simulink subsystem "template_MPC_offline_traj_shared_subsystem_MCP2_opti_qrqp"  (R2023b)
settings: Solver=VariableStepAuto  StartTime=0.0  StopTime=10.0  RelTol=1e-3
undefined symbols (not defined in the file): param_MPC2_qrqp_opti, param_MPC2_qrqp_opti_traj_data, param_weight_MPC2_qrqp_opti
settings Model: Creator=emu  LastModifiedBy=emu

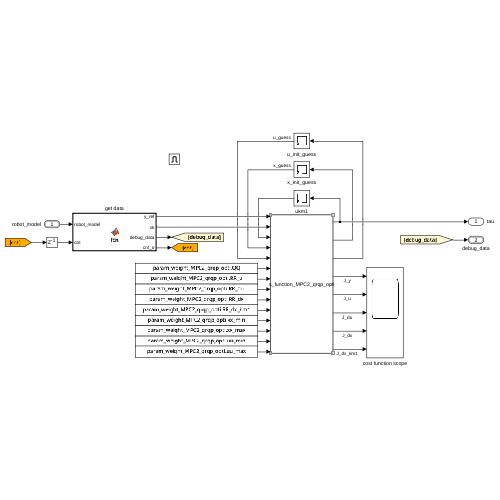
[thumbnail: Simulink's stored preview of the top-level diagram]
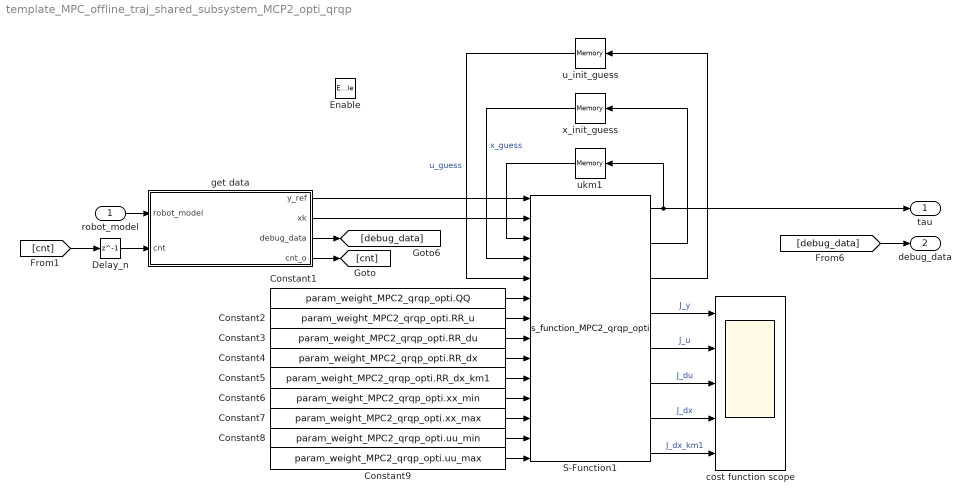
== system template_MPC_offline_traj_shared_subsystem_MCP2_opti_qrqp ==
  robot_model : Inport  OutDataTypeStr=Bus: robot_model
  Enable : EnablePort
  Constant1 : Constant  Value=param_weight_MPC2_qrqp_opti.QQ
  Constant2 : Constant  Value=param_weight_MPC2_qrqp_opti.RR_u
  Constant3 : Constant  Value=param_weight_MPC2_qrqp_opti.RR_du
  Constant4 : Constant  Value=param_weight_MPC2_qrqp_opti.RR_dx
  Constant5 : Constant  Value=param_weight_MPC2_qrqp_opti.RR_dx_km1
  Constant6 : Constant  Value=param_weight_MPC2_qrqp_opti.xx_min
  Constant7 : Constant  Value=param_weight_MPC2_qrqp_opti.xx_max
  Constant8 : Constant  Value=param_weight_MPC2_qrqp_opti.uu_min
  Constant9 : Constant  Value=param_weight_MPC2_qrqp_opti.uu_max
  Delay_n : Delay  DelayLength=1  InitialCondition=1
  S-Function1 : S-Function  FunctionName=s_function_MPC2_qrqp_opti  SFunctionModules='MPC2_qrqp_opti'  SFunctionDeploymentMode=off  EnableBusSupport=off
  cost function scope : Scope  NumInputPorts=5
  get data : MATLAB Function  TreatAsAtomicUnit=on
  u_init_guess : Memory  InitialCondition=param_MPC2_qrqp_opti.u_init_guess
  ukm1 : Memory  InitialCondition=param_MPC2_qrqp_opti.u_init_guess(:,1)
  x_init_guess : Memory  InitialCondition=param_MPC2_qrqp_opti.x_init_guess
  tau : Outport
  debug_data : Outport  Port=2  OutDataTypeStr=Bus: debug_data_bus
  wires:
  get data/1(y_ref) -> S-Function1/1
  S-Function1/6 -> cost function scope/3  "J_du"
  S-Function1/1 -> ukm1/1, tau/1
  ukm1/1 -> S-Function1/3
  x_init_guess/1 -> S-Function1/4  "x_guess"
  S-Function1/2 -> x_init_guess/1
  S-Function1/8 -> cost function scope/5  "J_dx_km1"
  S-Function1/3 -> u_init_guess/1
  get data/2(xk) -> S-Function1/2
  Constant4/1 -> S-Function1/9
  [cnt] -> Delay_n/1
  get data/4(cnt_o) -> [cnt]
  S-Function1/4 -> cost function scope/1  "J_y"
  Constant6/1 -> S-Function1/11
  S-Function1/5 -> cost function scope/2  "J_u"
  [debug_data] -> debug_data/1
  Constant9/1 -> S-Function1/14
  Delay_n/1 -> get data/2(cnt)
  u_init_guess/1 -> S-Function1/5  "u_guess"
  Constant8/1 -> S-Function1/13
  Constant3/1 -> S-Function1/8
  Constant5/1 -> S-Function1/10
  Constant2/1 -> S-Function1/7
  Constant1/1 -> S-Function1/6
  S-Function1/7 -> cost function scope/4  "J_dx"
  robot_model/1 -> get data/1(robot_model)
  get data/3(debug_data) -> [debug_data]
  Constant7/1 -> S-Function1/12

== matlab function template_MPC_offline_traj_shared_subsystem_MCP2_opti_qrqp/get data ==
  settings: updateMethod=DISCRETE  sampleTime=param_global.Ta
  data: y_ref output; robot_model input Bus: robot_model; cnt input; param_MPC2_qrqp_opti parameter; xk output; debug_data output Bus: debug_data_bus; cnt_o output; param_MPC2_qrqp_opti_traj_data parameter
function [y_ref, xk, debug_data, cnt_o] = fcn(robot_model, cnt, param_MPC2_qrqp_opti, param_MPC2_qrqp_opti_traj_data)

param_MPC = param_MPC2_qrqp_opti;
param_trajectory = param_MPC2_qrqp_opti_traj_data;

% Parameters
q = robot_model.q;      % generalized coordinates
q_p = robot_model.q_p;  % time derivative of generalized coordinates
H = robot_model.H;

% Current Pose of Endeffector
p = H(1:3,4);
R = H(1:3,1:3);

% desired Orientation as Rotationmatrix
q_e = rotation2quaternion(R);

% Error of Position (translation) and first time derivative
q_err = quat_mult(q_e, quat_inv(param_trajectory.q_d(cnt,:)));


xk = [q;q_p];

% Assemble vector of recieved output measurements
%y_ref = param_trajectory.p_d(i : param_MPC.N_step : i+ param_MPC.N * param_MPC.N_step, 1:2)';
p_d_traj = param_trajectory.p_d(cnt : param_MPC.N_step : cnt+ param_MPC.N * param_MPC.N_step, 1:3);
y_ref = p_d_traj(:, 1:2)';

cnt_o = cnt+1;

%% DEBUG
debug_data.x = p(1);
debug_data.x_d = y_ref(1,1);
debug_data.y =  p(2);
debug_data.y_d = y_ref(2,1);
debug_data.z =  p(3);
debug_data.z_d = p_d_traj(1,3);
debug_data.rot_x_err = q_err(2);
debug_data.rot_y_err = q_err(3);
debug_data.rot_z_err = q_err(4);
